simulink library "AEMS_Standard_Library"  (R2016b)
settings: Solver=ode45  StartTime=0.0  StopTime=10.0  RelTol=1e-3
undefined symbols (not defined in the file or in its folder): BkPY, carto, Cbx_extegr, Cbx_lpegrsys, Cbx_portegr, Cnx_bnk_nr_conf, Cnx_cyl_nr_conf, ConfigManagement, configuration_management, Cxx_dcm_io_tmr_end_xxxx, Cxx_dcm_rt_tmr_end, Cxx_DID_xxxx_IO_max, Cxx_DID_xxxx_IO_min, Cxx_egrhsofs, Cxx_vmaniegi, DEM_DEBOUNCE_FREEZE, DEM_DTR_CTL_INVISIBLE, DEM_DTR_CTL_NORMAL, Dem_DtrId2_XXX, Dem_DtrId3_XXX, Dem_DtrId4_XXX, Dem_DtrId5_XXX, Dem_DtrId6_XXX, Dem_DtrId7_XXX, Dem_DtrId8_XXX, Dem_DtrId9_XXX, Dem_DtrId_XXX, Dem_EnableConditionId2_XXX, Dem_EnableConditionId3_XXX, Dem_EnableConditionId4_XXX, Dem_EnableConditionId5_XXX, Dem_EnableConditionId6_XXX, Dem_EnableConditionId7_XXX, Dem_EnableConditionId8_XXX, Dem_EnableConditionId_XXX, Dem_EventId, Dem_EventId2_XXX, Dem_EventId3_XXX, Dem_EventId4_XXX, Dem_EventId5_XXX, Dem_EventId6_XXX, Dem_EventId7_XXX, Dem_EventId8_XXX, Dem_EventId9_XXX, Dem_EventId_Device_Faulttype, Dem_EventId_XXX, DEM_IUMPR_GENERAL_DENOMINATOR, DEM_OPCYC_IGNITION, Dem_RatioId2_XXX, Dem_RatioId3_XXX, Dem_RatioId4_XXX, Dem_RatioId5_XXX, Dem_RatioId6_XXX, Dem_RatioId7_XXX, Dem_RatioId8_XXX, Dem_RatioId_XXX, Dem_StorageConditionId2_XXX, Dem_StorageConditionId3_XXX, Dem_StorageConditionId4_XXX, Dem_StorageConditionId5_XXX ... (+65)
libraries: AEMS_Standard_Library x477, simulink x2
(part 32 of 39)

== system AEMS_Standard_Library/SUB/AEMS_DEM_SET_DTR_2DU/Dem_SetDTR_Call1 ==
  testresult1 : Inport  Interpolate=off
  lowerlimit1 : Inport  Port=2  Interpolate=off
  upperlimit1 : Inport  Port=3  Interpolate=off
  ctrl_flag1 : Inport  Port=4  Interpolate=off
  set_flag1 : EnablePort
      settings: AttributesFormatString=<states=%<StatesWhenEnabling>>
  AEMS_DEM_SETDTR1 : AEMS_Standard_Library/SUB/AEMS_DEM_SETDTR
      settings: AttributesFormatString=%<MaskType>
  Ctrlval_block1 : Constant  Value=DEM_DTR_CTL_NORMAL  OutDataTypeStr=uint8
  Ctrlval_block2 : Constant  Value=DEM_DTR_CTL_INVISIBLE  OutDataTypeStr=uint8
  DTRId_block1 : Constant  Value=Dem_DtrId_XXX  OutDataTypeStr=uint16
  Data Type Conversion : DataTypeConversion  OutDataTypeStr=int32  SaturateOnIntegerOverflow=on
  Data Type Conversion1 : DataTypeConversion  OutDataTypeStr=int32  SaturateOnIntegerOverflow=on
  Data Type Conversion2 : DataTypeConversion  OutDataTypeStr=int32  SaturateOnIntegerOverflow=on
  Limitter1 : Saturate  UpperLimit=1  LowerLimit=0
      settings: AttributesFormatString=<limits=%<UpperLimit>/%<LowerLimit>>
  Limitter2 : Saturate  UpperLimit=1  LowerLimit=0
      settings: AttributesFormatString=<limits=%<UpperLimit>/%<LowerLimit>>
  Limitter3 : Saturate  UpperLimit=1  LowerLimit=0
      settings: AttributesFormatString=<limits=%<UpperLimit>/%<LowerLimit>>
  Sum : Sum  OutDataTypeStr=Inherit: Inherit via back propagation  SaturateOnIntegerOverflow=on  InputSameDT=on
  Sum1 : Sum  OutDataTypeStr=Inherit: Inherit via back propagation  SaturateOnIntegerOverflow=on  InputSameDT=on
  Sum2 : Sum  OutDataTypeStr=Inherit: Inherit via back propagation  SaturateOnIntegerOverflow=on  InputSameDT=on
  Switch : Switch  Criteria=u2 ~= 0  ZeroCross=off  InputSameDT=on
      settings: AttributesFormatString=Criteria=%<Criteria>
  offset1 : Constant  Value=0  OutDataTypeStr=uint16
  offset2 : Constant  Value=0  OutDataTypeStr=uint16
  offset3 : Constant  Value=0  OutDataTypeStr=uint16
  wires:
  Switch/1 -> AEMS_DEM_SETDTR1/5  "ctrlval1"
  Ctrlval_block2/1 -> Switch/3
  ctrl_flag1/1 -> Switch/2
  Ctrlval_block1/1 -> Switch/1
  offset1/1 -> Sum/1
  Limitter1/1 -> Sum/2
  offset2/1 -> Sum1/1
  Limitter2/1 -> Sum1/2
  offset3/1 -> Sum2/1
  Limitter3/1 -> Sum2/2
  Sum/1 -> Data Type Conversion/1
  Sum1/1 -> Data Type Conversion1/1
  Sum2/1 -> Data Type Conversion2/1
  testresult1/1 -> Limitter1/1
  lowerlimit1/1 -> Limitter2/1
  upperlimit1/1 -> Limitter3/1
  Data Type Conversion/1 -> AEMS_DEM_SETDTR1/2  "result1"
  DTRId_block1/1 -> AEMS_DEM_SETDTR1/1  "dtrid1"
  Data Type Conversion1/1 -> AEMS_DEM_SETDTR1/3  "lowlimit1"
  Data Type Conversion2/1 -> AEMS_DEM_SETDTR1/4  "uplimit1"

== system AEMS_Standard_Library/SUB/AEMS_DEM_SET_DTR_2DU/Dem_SetDTR_Call2 ==
  testresult2 : Inport  Interpolate=off
  lowerlimit2 : Inport  Port=2  Interpolate=off
  upperlimit2 : Inport  Port=3  Interpolate=off
  ctrl_flag2 : Inport  Port=4  Interpolate=off
  set_flag2 : EnablePort
      settings: AttributesFormatString=<states=%<StatesWhenEnabling>>
  AEMS_DEM_SETDTR2 : AEMS_Standard_Library/SUB/AEMS_DEM_SETDTR
      settings: AttributesFormatString=%<MaskType>
  Ctrlval_block1 : Constant  Value=DEM_DTR_CTL_NORMAL  OutDataTypeStr=uint8
  Ctrlval_block2 : Constant  Value=DEM_DTR_CTL_INVISIBLE  OutDataTypeStr=uint8
  DTRId_block2 : Constant  Value=Dem_DtrId2_XXX  OutDataTypeStr=uint16
  Data Type Conversion3 : DataTypeConversion  OutDataTypeStr=int32  SaturateOnIntegerOverflow=on
  Data Type Conversion4 : DataTypeConversion  OutDataTypeStr=int32  SaturateOnIntegerOverflow=on
  Data Type Conversion5 : DataTypeConversion  OutDataTypeStr=int32  SaturateOnIntegerOverflow=on
  Limitter4 : Saturate  UpperLimit=1  LowerLimit=0
      settings: AttributesFormatString=<limits=%<UpperLimit>/%<LowerLimit>>
  Limitter5 : Saturate  UpperLimit=1  LowerLimit=0
      settings: AttributesFormatString=<limits=%<UpperLimit>/%<LowerLimit>>
  Limitter6 : Saturate  UpperLimit=1  LowerLimit=0
      settings: AttributesFormatString=<limits=%<UpperLimit>/%<LowerLimit>>
  Sum3 : Sum  OutDataTypeStr=Inherit: Inherit via back propagation  SaturateOnIntegerOverflow=on  InputSameDT=on
  Sum4 : Sum  OutDataTypeStr=Inherit: Inherit via back propagation  SaturateOnIntegerOverflow=on  InputSameDT=on
  Sum5 : Sum  OutDataTypeStr=Inherit: Inherit via back propagation  SaturateOnIntegerOverflow=on  InputSameDT=on
  Switch : Switch  Criteria=u2 ~= 0  ZeroCross=off  InputSameDT=on
      settings: AttributesFormatString=Criteria=%<Criteria>
  offset4 : Constant  Value=0  OutDataTypeStr=uint16
  offset5 : Constant  Value=0  OutDataTypeStr=uint16
  offset6 : Constant  Value=0  OutDataTypeStr=uint16
  wires:
  Ctrlval_block1/1 -> Switch/1
  Switch/1 -> AEMS_DEM_SETDTR2/5  "ctrlval2"
  Ctrlval_block2/1 -> Switch/3
  ctrl_flag2/1 -> Switch/2
  offset4/1 -> Sum3/1
  Limitter4/1 -> Sum3/2
  offset5/1 -> Sum4/1
  Limitter5/1 -> Sum4/2
  offset6/1 -> Sum5/1
  Limitter6/1 -> Sum5/2
  Sum3/1 -> Data Type Conversion3/1
  Sum4/1 -> Data Type Conversion4/1
  Sum5/1 -> Data Type Conversion5/1
  testresult2/1 -> Limitter4/1
  lowerlimit2/1 -> Limitter5/1
  upperlimit2/1 -> Limitter6/1
  DTRId_block2/1 -> AEMS_DEM_SETDTR2/1  "dtrid2"
  Data Type Conversion3/1 -> AEMS_DEM_SETDTR2/2  "result2"
  Data Type Conversion4/1 -> AEMS_DEM_SETDTR2/3  "lowlimit2"
  Data Type Conversion5/1 -> AEMS_DEM_SETDTR2/4  "uplimit2"

== system AEMS_Standard_Library/SUB/AEMS_DEM_SET_DTR_8DS/Deadzone ==
  testresult : Inport  Interpolate=off
  lowerlimit : Inport  Port=2  Interpolate=off
  upperlimit : Inport  Port=3  Interpolate=off
  Sum1 : Sum  Inputs=-+  OutDataTypeStr=Inherit: Inherit via back propagation  InputSameDT=on
  Sum3 : Sum  OutDataTypeStr=Inherit: Inherit via back propagation  SaturateOnIntegerOverflow=on  InputSameDT=on
  Switch{,1,3..4} (4 alike) : Switch  Criteria=u2 ~= 0  ZeroCross=off  InputSameDT=on
      settings: AttributesFormatString=Criteria=%<Criteria>
  relational2 : RelationalOperator  DisableCoverage=on  OutDataTypeStr=boolean  ZeroCross=off  RndMeth=Nearest  InputSameDT=on
  relational3 : RelationalOperator  DisableCoverage=on  Operator=<  OutDataTypeStr=boolean  ZeroCross=off  RndMeth=Nearest  InputSameDT=on
  relational4 : RelationalOperator  DisableCoverage=on  OutDataTypeStr=boolean  ZeroCross=off  RndMeth=Nearest  InputSameDT=on
  relational5 : RelationalOperator  DisableCoverage=on  Operator=<=  OutDataTypeStr=boolean  ZeroCross=off  RndMeth=Nearest  InputSameDT=on
  resolution_block1 : Constant  OutDataTypeStr=single
  resolution_block2 : Constant  OutDataTypeStr=single
  customresult : Outport
  wires:
  Switch/1 -> customresult/1  "customresult"
  Sum3/1 -> Switch1/1, relational2/2
  Switch4/1 -> Switch3/3
  Switch1/1 -> Switch/3
  lowerlimit/1 -> relational4/2, Sum1/2
  relational5/1 -> Switch4/2
  relational4/1 -> Switch3/2
  relational3/1 -> Switch1/2
  resolution_block1/1 -> Sum3/2
  upperlimit/1 -> Sum3/1, relational3/1
  relational2/1 -> Switch/2
  testresult/1 -> Switch/1, relational2/1, relational4/1, Switch3/1, Switch4/3, relational5/2, relational3/2
  Switch3/1 -> Switch1/3
  Sum1/1 -> relational5/1, Switch4/1
  resolution_block2/1 -> Sum1/1

== system AEMS_Standard_Library/SUB/AEMS_DEM_SET_DTR_8DS/Dem_SetDTR_Call1 ==
  customresult1 : Inport  Interpolate=off
  lowerlimit1 : Inport  Port=2  Interpolate=off
  upperlimit1 : Inport  Port=3  Interpolate=off
  ctrl_flag1 : Inport  Port=4  Interpolate=off
  set_flag1 : EnablePort
      settings: AttributesFormatString=<states=%<StatesWhenEnabling>>
  AEMS_DEM_SETDTR1 : AEMS_Standard_Library/SUB/AEMS_DEM_SETDTR  Tag=[LIB]
      settings: AttributesFormatString=%<MaskType>
  Ctrlval_block1 : Constant  Value=DEM_DTR_CTL_NORMAL  OutDataTypeStr=uint8
  Ctrlval_block2 : Constant  Value=DEM_DTR_CTL_INVISIBLE  OutDataTypeStr=uint8
  DTRId_block1 : Constant  Value=Dem_DtrId_XXX  OutDataTypeStr=uint16
  Data Type Conversion : DataTypeConversion  OutDataTypeStr=int32  SaturateOnIntegerOverflow=on
  Data Type Conversion1 : DataTypeConversion  OutDataTypeStr=int32  SaturateOnIntegerOverflow=on
  Data Type Conversion2 : DataTypeConversion  OutDataTypeStr=int32  SaturateOnIntegerOverflow=on
  Divide1 : Product  Inputs=*/  OutDataTypeStr=Inherit: Inherit via back propagation  SaturateOnIntegerOverflow=on
  Divide2 : Product  Inputs=*/  OutDataTypeStr=Inherit: Inherit via back propagation  SaturateOnIntegerOverflow=on
  Divide3 : Product  Inputs=*/  OutDataTypeStr=Inherit: Inherit via back propagation  SaturateOnIntegerOverflow=on
  Limitter1 : Saturate  UpperLimit=1  LowerLimit=0
      settings: AttributesFormatString=<limits=%<UpperLimit>/%<LowerLimit>>
  Limitter2 : Saturate  UpperLimit=1  LowerLimit=0
      settings: AttributesFormatString=<limits=%<UpperLimit>/%<LowerLimit>>
  Limitter3 : Saturate  UpperLimit=1  LowerLimit=0
      settings: AttributesFormatString=<limits=%<UpperLimit>/%<LowerLimit>>
  Resolution_block1 : Constant  OutDataTypeStr=single
  Resolution_block2 : Constant  OutDataTypeStr=single
  Resolution_block3 : Constant  OutDataTypeStr=single
  Switch : Switch  Criteria=u2 ~= 0  ZeroCross=off  InputSameDT=on
      settings: AttributesFormatString=Criteria=%<Criteria>
  wires:
  DTRId_block1/1 -> AEMS_DEM_SETDTR1/1  "dtrid1"
  Resolution_block1/1 -> Divide1/2
  Limitter1/1 -> Divide1/1
  Limitter3/1 -> Divide3/1
  customresult1/1 -> Limitter1/1
  lowerlimit1/1 -> Limitter2/1
  upperlimit1/1 -> Limitter3/1
  Data Type Conversion1/1 -> AEMS_DEM_SETDTR1/3  "lowlimit1"
  Data Type Conversion2/1 -> AEMS_DEM_SETDTR1/4  "uplimit1"
  Data Type Conversion/1 -> AEMS_DEM_SETDTR1/2  "result1"
  Limitter2/1 -> Divide2/1
  Resolution_block2/1 -> Divide2/2
  Resolution_block3/1 -> Divide3/2
  Switch/1 -> AEMS_DEM_SETDTR1/5  "ctrlval1"
  Ctrlval_block1/1 -> Switch/1
  ctrl_flag1/1 -> Switch/2
  Ctrlval_block2/1 -> Switch/3
  Divide1/1 -> Data Type Conversion/1
  Divide2/1 -> Data Type Conversion1/1
  Divide3/1 -> Data Type Conversion2/1

== system AEMS_Standard_Library/SUB/AEMS_DEM_SET_DTR_8DS/Dem_SetDTR_Call2 ==
  customresult2 : Inport  Interpolate=off
  lowerlimit2 : Inport  Port=2  Interpolate=off
  upperlimit2 : Inport  Port=3  Interpolate=off
  ctrl_flag2 : Inport  Port=4  Interpolate=off
  set_flag2 : EnablePort
      settings: AttributesFormatString=<states=%<StatesWhenEnabling>>
  AEMS_DEM_SETDTR2 : AEMS_Standard_Library/SUB/AEMS_DEM_SETDTR  Tag=[LIB]
      settings: AttributesFormatString=%<MaskType>
  Ctrlval_block1 : Constant  Value=DEM_DTR_CTL_NORMAL  OutDataTypeStr=uint8
  Ctrlval_block2 : Constant  Value=DEM_DTR_CTL_INVISIBLE  OutDataTypeStr=uint8
  DTRId_block2 : Constant  Value=Dem_DtrId2_XXX  OutDataTypeStr=uint16
  Data Type Conversion : DataTypeConversion  OutDataTypeStr=int32  SaturateOnIntegerOverflow=on
  Data Type Conversion1 : DataTypeConversion  OutDataTypeStr=int32  SaturateOnIntegerOverflow=on
  Data Type Conversion2 : DataTypeConversion  OutDataTypeStr=int32  SaturateOnIntegerOverflow=on
  Divide1 : Product  Inputs=*/  OutDataTypeStr=Inherit: Inherit via back propagation  SaturateOnIntegerOverflow=on
  Divide2 : Product  Inputs=*/  OutDataTypeStr=Inherit: Inherit via back propagation  SaturateOnIntegerOverflow=on
  Divide3 : Product  Inputs=*/  OutDataTypeStr=Inherit: Inherit via back propagation  SaturateOnIntegerOverflow=on
  Limitter4 : Saturate  UpperLimit=1  LowerLimit=0
      settings: AttributesFormatString=<limits=%<UpperLimit>/%<LowerLimit>>
  Limitter5 : Saturate  UpperLimit=1  LowerLimit=0
      settings: AttributesFormatString=<limits=%<UpperLimit>/%<LowerLimit>>
  Limitter6 : Saturate  UpperLimit=1  LowerLimit=0
      settings: AttributesFormatString=<limits=%<UpperLimit>/%<LowerLimit>>
  Resolution_block4 : Constant  OutDataTypeStr=single
  Resolution_block5 : Constant  OutDataTypeStr=single
  Resolution_block6 : Constant  OutDataTypeStr=single
  Switch : Switch  Criteria=u2 ~= 0  ZeroCross=off  InputSameDT=on
      settings: AttributesFormatString=Criteria=%<Criteria>
  wires:
  DTRId_block2/1 -> AEMS_DEM_SETDTR2/1  "dtrid2"
  Resolution_block4/1 -> Divide1/2
  Limitter4/1 -> Divide1/1
  Limitter6/1 -> Divide3/1
  customresult2/1 -> Limitter4/1
  lowerlimit2/1 -> Limitter5/1
  upperlimit2/1 -> Limitter6/1
  Data Type Conversion1/1 -> AEMS_DEM_SETDTR2/3  "lowlimit2"
  Data Type Conversion2/1 -> AEMS_DEM_SETDTR2/4  "uplimit2"
  Data Type Conversion/1 -> AEMS_DEM_SETDTR2/2  "result2"
  Limitter5/1 -> Divide2/1
  Resolution_block5/1 -> Divide2/2
  Resolution_block6/1 -> Divide3/2
  Divide1/1 -> Data Type Conversion/1
  Divide2/1 -> Data Type Conversion1/1
  Divide3/1 -> Data Type Conversion2/1
  Switch/1 -> AEMS_DEM_SETDTR2/5  "ctrlval2"
  Ctrlval_block1/1 -> Switch/1
  ctrl_flag2/1 -> Switch/2
  Ctrlval_block2/1 -> Switch/3

== system AEMS_Standard_Library/SUB/AEMS_DEM_SET_DTR_8DS/Dem_SetDTR_Call3 ==
  customresult3 : Inport  Interpolate=off
  lowerlimit3 : Inport  Port=2  Interpolate=off
  upperlimit3 : Inport  Port=3  Interpolate=off
  ctrl_flag3 : Inport  Port=4  Interpolate=off
  set_flag3 : EnablePort
      settings: AttributesFormatString=<states=%<StatesWhenEnabling>>
  AEMS_DEM_SETDTR3 : AEMS_Standard_Library/SUB/AEMS_DEM_SETDTR  Tag=[LIB]
      settings: AttributesFormatString=%<MaskType>
  Ctrlval_block1 : Constant  Value=DEM_DTR_CTL_NORMAL  OutDataTypeStr=uint8
  Ctrlval_block2 : Constant  Value=DEM_DTR_CTL_INVISIBLE  OutDataTypeStr=uint8
  DTRId_block3 : Constant  Value=Dem_DtrId3_XXX  OutDataTypeStr=uint16
  Data Type Conversion : DataTypeConversion  OutDataTypeStr=int32  SaturateOnIntegerOverflow=on
  Data Type Conversion1 : DataTypeConversion  OutDataTypeStr=int32  SaturateOnIntegerOverflow=on
  Data Type Conversion2 : DataTypeConversion  OutDataTypeStr=int32  SaturateOnIntegerOverflow=on
  Divide1 : Product  Inputs=*/  OutDataTypeStr=Inherit: Inherit via back propagation  SaturateOnIntegerOverflow=on
  Divide2 : Product  Inputs=*/  OutDataTypeStr=Inherit: Inherit via back propagation  SaturateOnIntegerOverflow=on
  Divide3 : Product  Inputs=*/  OutDataTypeStr=Inherit: Inherit via back propagation  SaturateOnIntegerOverflow=on
  Limitter7 : Saturate  UpperLimit=1  LowerLimit=0
      settings: AttributesFormatString=<limits=%<UpperLimit>/%<LowerLimit>>
  Limitter8 : Saturate  UpperLimit=1  LowerLimit=0
      settings: AttributesFormatString=<limits=%<UpperLimit>/%<LowerLimit>>
  Limitter9 : Saturate  UpperLimit=1  LowerLimit=0
      settings: AttributesFormatString=<limits=%<UpperLimit>/%<LowerLimit>>
  Resolution_block7 : Constant  OutDataTypeStr=single
  Resolution_block8 : Constant  OutDataTypeStr=single
  Resolution_block9 : Constant  OutDataTypeStr=single
  Switch : Switch  Criteria=u2 ~= 0  ZeroCross=off  InputSameDT=on
      settings: AttributesFormatString=Criteria=%<Criteria>
  wires:
  DTRId_block3/1 -> AEMS_DEM_SETDTR3/1  "dtrid3"
  Resolution_block7/1 -> Divide1/2
  Limitter7/1 -> Divide1/1
  Limitter9/1 -> Divide3/1
  customresult3/1 -> Limitter7/1
  lowerlimit3/1 -> Limitter8/1
  upperlimit3/1 -> Limitter9/1
  Data Type Conversion1/1 -> AEMS_DEM_SETDTR3/3  "lowlimit3"
  Data Type Conversion2/1 -> AEMS_DEM_SETDTR3/4  "uplimit3"
  Data Type Conversion/1 -> AEMS_DEM_SETDTR3/2  "result3"
  Limitter8/1 -> Divide2/1
  Resolution_block8/1 -> Divide2/2
  Resolution_block9/1 -> Divide3/2
  Divide1/1 -> Data Type Conversion/1
  Divide2/1 -> Data Type Conversion1/1
  Divide3/1 -> Data Type Conversion2/1
  Switch/1 -> AEMS_DEM_SETDTR3/5  "ctrlval3"
  Ctrlval_block1/1 -> Switch/1
  ctrl_flag3/1 -> Switch/2
  Ctrlval_block2/1 -> Switch/3

== system AEMS_Standard_Library/SUB/AEMS_DEM_SET_DTR_8DS/Dem_SetDTR_Call4 ==
  customresult4 : Inport  Interpolate=off
  lowerlimit4 : Inport  Port=2  Interpolate=off
  upperlimit4 : Inport  Port=3  Interpolate=off
  ctrl_flag4 : Inport  Port=4  Interpolate=off
  set_flag4 : EnablePort
      settings: AttributesFormatString=<states=%<StatesWhenEnabling>>
  AEMS_DEM_SETDTR4 : AEMS_Standard_Library/SUB/AEMS_DEM_SETDTR  Tag=[LIB]
      settings: AttributesFormatString=%<MaskType>
  Ctrlval_block1 : Constant  Value=DEM_DTR_CTL_NORMAL  OutDataTypeStr=uint8
  Ctrlval_block2 : Constant  Value=DEM_DTR_CTL_INVISIBLE  OutDataTypeStr=uint8
  DTRId_block4 : Constant  Value=Dem_DtrId4_XXX  OutDataTypeStr=uint16
  Data Type Conversion : DataTypeConversion  OutDataTypeStr=int32  SaturateOnIntegerOverflow=on
  Data Type Conversion1 : DataTypeConversion  OutDataTypeStr=int32  SaturateOnIntegerOverflow=on
  Data Type Conversion2 : DataTypeConversion  OutDataTypeStr=int32  SaturateOnIntegerOverflow=on
  Divide1 : Product  Inputs=*/  OutDataTypeStr=Inherit: Inherit via back propagation  SaturateOnIntegerOverflow=on
  Divide2 : Product  Inputs=*/  OutDataTypeStr=Inherit: Inherit via back propagation  SaturateOnIntegerOverflow=on
  Divide3 : Product  Inputs=*/  OutDataTypeStr=Inherit: Inherit via back propagation  SaturateOnIntegerOverflow=on
  Limitter10 : Saturate  UpperLimit=1  LowerLimit=0
      settings: AttributesFormatString=<limits=%<UpperLimit>/%<LowerLimit>>
  Limitter11 : Saturate  UpperLimit=1  LowerLimit=0
      settings: AttributesFormatString=<limits=%<UpperLimit>/%<LowerLimit>>
  Limitter12 : Saturate  UpperLimit=1  LowerLimit=0
      settings: AttributesFormatString=<limits=%<UpperLimit>/%<LowerLimit>>
  Resolution_block10 : Constant  OutDataTypeStr=single
  Resolution_block11 : Constant  OutDataTypeStr=single
  Resolution_block12 : Constant  OutDataTypeStr=single
  Switch : Switch  Criteria=u2 ~= 0  ZeroCross=off  InputSameDT=on
      settings: AttributesFormatString=Criteria=%<Criteria>
  wires:
  DTRId_block4/1 -> AEMS_DEM_SETDTR4/1  "dtrid4"
  Resolution_block10/1 -> Divide1/2
  Limitter10/1 -> Divide1/1
  Limitter12/1 -> Divide3/1
  customresult4/1 -> Limitter10/1
  lowerlimit4/1 -> Limitter11/1
  upperlimit4/1 -> Limitter12/1
  Data Type Conversion1/1 -> AEMS_DEM_SETDTR4/3  "lowlimit4"
  Data Type Conversion2/1 -> AEMS_DEM_SETDTR4/4  "uplimit4"
  Data Type Conversion/1 -> AEMS_DEM_SETDTR4/2  "result4"
  Limitter11/1 -> Divide2/1
  Resolution_block11/1 -> Divide2/2
  Resolution_block12/1 -> Divide3/2
  Ctrlval_block1/1 -> Switch/1
  ctrl_flag4/1 -> Switch/2
  Ctrlval_block2/1 -> Switch/3
  Switch/1 -> AEMS_DEM_SETDTR4/5  "ctrlval4"
  Divide3/1 -> Data Type Conversion2/1
  Divide2/1 -> Data Type Conversion1/1
  Divide1/1 -> Data Type Conversion/1

== system AEMS_Standard_Library/SUB/AEMS_DEM_SET_DTR_8DS/Dem_SetDTR_Call5 ==
  customresult5 : Inport  Interpolate=off
  lowerlimit5 : Inport  Port=2  Interpolate=off
  upperlimit5 : Inport  Port=3  Interpolate=off
  ctrl_flag5 : Inport  Port=4  Interpolate=off
  set_flag5 : EnablePort
      settings: AttributesFormatString=<states=%<StatesWhenEnabling>>
  AEMS_DEM_SETDTR5 : AEMS_Standard_Library/SUB/AEMS_DEM_SETDTR  Tag=[LIB]
      settings: AttributesFormatString=%<MaskType>
  Ctrlval_block1 : Constant  Value=DEM_DTR_CTL_NORMAL  OutDataTypeStr=uint8
  Ctrlval_block2 : Constant  Value=DEM_DTR_CTL_INVISIBLE  OutDataTypeStr=uint8
  DTRId_block5 : Constant  Value=Dem_DtrId5_XXX  OutDataTypeStr=uint16
  Data Type Conversion : DataTypeConversion  OutDataTypeStr=int32  SaturateOnIntegerOverflow=on
  Data Type Conversion1 : DataTypeConversion  OutDataTypeStr=int32  SaturateOnIntegerOverflow=on
  Data Type Conversion2 : DataTypeConversion  OutDataTypeStr=int32  SaturateOnIntegerOverflow=on
  Divide1 : Product  Inputs=*/  OutDataTypeStr=Inherit: Inherit via back propagation  SaturateOnIntegerOverflow=on
  Divide2 : Product  Inputs=*/  OutDataTypeStr=Inherit: Inherit via back propagation  SaturateOnIntegerOverflow=on
  Divide3 : Product  Inputs=*/  OutDataTypeStr=Inherit: Inherit via back propagation  SaturateOnIntegerOverflow=on
  Limitter13 : Saturate  UpperLimit=1  LowerLimit=0
      settings: AttributesFormatString=<limits=%<UpperLimit>/%<LowerLimit>>
  Limitter14 : Saturate  UpperLimit=1  LowerLimit=0
      settings: AttributesFormatString=<limits=%<UpperLimit>/%<LowerLimit>>
  Limitter15 : Saturate  UpperLimit=1  LowerLimit=0
      settings: AttributesFormatString=<limits=%<UpperLimit>/%<LowerLimit>>
  Resolution_block13 : Constant  OutDataTypeStr=single
  Resolution_block14 : Constant  OutDataTypeStr=single
  Resolution_block15 : Constant  OutDataTypeStr=single
  Switch : Switch  Criteria=u2 ~= 0  ZeroCross=off  InputSameDT=on
      settings: AttributesFormatString=Criteria=%<Criteria>
  wires:
  DTRId_block5/1 -> AEMS_DEM_SETDTR5/1  "dtrid5"
  Resolution_block13/1 -> Divide1/2
  Limitter13/1 -> Divide1/1
  Limitter15/1 -> Divide3/1
  customresult5/1 -> Limitter13/1
  lowerlimit5/1 -> Limitter14/1
  upperlimit5/1 -> Limitter15/1
  Data Type Conversion1/1 -> AEMS_DEM_SETDTR5/3  "lowlimit5"
  Switch/1 -> AEMS_DEM_SETDTR5/5  "ctrlval5"
  Data Type Conversion2/1 -> AEMS_DEM_SETDTR5/4  "uplimit5"
  Data Type Conversion/1 -> AEMS_DEM_SETDTR5/2  "result5"
  Limitter14/1 -> Divide2/1
  Resolution_block14/1 -> Divide2/2
  Resolution_block15/1 -> Divide3/2
  Divide1/1 -> Data Type Conversion/1
  Divide2/1 -> Data Type Conversion1/1
  Divide3/1 -> Data Type Conversion2/1
  Ctrlval_block1/1 -> Switch/1
  ctrl_flag5/1 -> Switch/2
  Ctrlval_block2/1 -> Switch/3

== system AEMS_Standard_Library/SUB/AEMS_DEM_SET_DTR_8DS/Dem_SetDTR_Call6 ==
  customresult6 : Inport  Interpolate=off
  lowerlimit6 : Inport  Port=2  Interpolate=off
  upperlimit6 : Inport  Port=3  Interpolate=off
  ctrl_flag6 : Inport  Port=4  Interpolate=off
  set_flag6 : EnablePort
      settings: AttributesFormatString=<states=%<StatesWhenEnabling>>
  AEMS_DEM_SETDTR6 : AEMS_Standard_Library/SUB/AEMS_DEM_SETDTR  Tag=[LIB]
      settings: AttributesFormatString=%<MaskType>
  Ctrlval_block1 : Constant  Value=DEM_DTR_CTL_NORMAL  OutDataTypeStr=uint8
  Ctrlval_block2 : Constant  Value=DEM_DTR_CTL_INVISIBLE  OutDataTypeStr=uint8
  DTRId_block6 : Constant  Value=Dem_DtrId6_XXX  OutDataTypeStr=uint16
  Data Type Conversion : DataTypeConversion  OutDataTypeStr=int32  SaturateOnIntegerOverflow=on
  Data Type Conversion1 : DataTypeConversion  OutDataTypeStr=int32  SaturateOnIntegerOverflow=on
  Data Type Conversion2 : DataTypeConversion  OutDataTypeStr=int32  SaturateOnIntegerOverflow=on
  Divide1 : Product  Inputs=*/  OutDataTypeStr=Inherit: Inherit via back propagation  SaturateOnIntegerOverflow=on
  Divide2 : Product  Inputs=*/  OutDataTypeStr=Inherit: Inherit via back propagation  SaturateOnIntegerOverflow=on
  Divide3 : Product  Inputs=*/  OutDataTypeStr=Inherit: Inherit via back propagation  SaturateOnIntegerOverflow=on
  Limitter16 : Saturate  UpperLimit=1  LowerLimit=0
      settings: AttributesFormatString=<limits=%<UpperLimit>/%<LowerLimit>>
  Limitter17 : Saturate  UpperLimit=1  LowerLimit=0
      settings: AttributesFormatString=<limits=%<UpperLimit>/%<LowerLimit>>
  Limitter18 : Saturate  UpperLimit=1  LowerLimit=0
      settings: AttributesFormatString=<limits=%<UpperLimit>/%<LowerLimit>>
  Resolution_block16 : Constant  OutDataTypeStr=single
  Resolution_block17 : Constant  OutDataTypeStr=single
  Resolution_block18 : Constant  OutDataTypeStr=single
  Switch : Switch  Criteria=u2 ~= 0  ZeroCross=off  InputSameDT=on
      settings: AttributesFormatString=Criteria=%<Criteria>
  wires:
  DTRId_block6/1 -> AEMS_DEM_SETDTR6/1  "dtrid6"
  Resolution_block16/1 -> Divide1/2
  Limitter16/1 -> Divide1/1
  Limitter18/1 -> Divide3/1
  customresult6/1 -> Limitter16/1
  lowerlimit6/1 -> Limitter17/1
  upperlimit6/1 -> Limitter18/1
  Data Type Conversion1/1 -> AEMS_DEM_SETDTR6/3  "lowlimit6"
  Switch/1 -> AEMS_DEM_SETDTR6/5  "ctrlval6"
  Data Type Conversion2/1 -> AEMS_DEM_SETDTR6/4  "uplimit6"
  Data Type Conversion/1 -> AEMS_DEM_SETDTR6/2  "result6"
  Limitter17/1 -> Divide2/1
  Resolution_block17/1 -> Divide2/2
  Resolution_block18/1 -> Divide3/2
  Ctrlval_block1/1 -> Switch/1
  ctrl_flag6/1 -> Switch/2
  Ctrlval_block2/1 -> Switch/3
  Divide3/1 -> Data Type Conversion2/1
  Divide2/1 -> Data Type Conversion1/1
  Divide1/1 -> Data Type Conversion/1

== system AEMS_Standard_Library/SUB/AEMS_DEM_SET_DTR_8DS/Dem_SetDTR_Call7 ==
  customresult7 : Inport  Interpolate=off
  lowerlimit7 : Inport  Port=2  Interpolate=off
  upperlimit7 : Inport  Port=3  Interpolate=off
  ctrl_flag7 : Inport  Port=4  Interpolate=off
  set_flag7 : EnablePort
      settings: AttributesFormatString=<states=%<StatesWhenEnabling>>
  AEMS_DEM_SETDTR7 : AEMS_Standard_Library/SUB/AEMS_DEM_SETDTR  Tag=[LIB]
      settings: AttributesFormatString=%<MaskType>
  Ctrlval_block1 : Constant  Value=DEM_DTR_CTL_NORMAL  OutDataTypeStr=uint8
  Ctrlval_block2 : Constant  Value=DEM_DTR_CTL_INVISIBLE  OutDataTypeStr=uint8
  DTRId_block7 : Constant  Value=Dem_DtrId7_XXX  OutDataTypeStr=uint16
  Data Type Conversion : DataTypeConversion  OutDataTypeStr=int32  SaturateOnIntegerOverflow=on
  Data Type Conversion1 : DataTypeConversion  OutDataTypeStr=int32  SaturateOnIntegerOverflow=on
  Data Type Conversion2 : DataTypeConversion  OutDataTypeStr=int32  SaturateOnIntegerOverflow=on
  Divide1 : Product  Inputs=*/  OutDataTypeStr=Inherit: Inherit via back propagation  SaturateOnIntegerOverflow=on
  Divide2 : Product  Inputs=*/  OutDataTypeStr=Inherit: Inherit via back propagation  SaturateOnIntegerOverflow=on
  Divide3 : Product  Inputs=*/  OutDataTypeStr=Inherit: Inherit via back propagation  SaturateOnIntegerOverflow=on
  Limitter19 : Saturate  UpperLimit=1  LowerLimit=0
      settings: AttributesFormatString=<limits=%<UpperLimit>/%<LowerLimit>>
  Limitter20 : Saturate  UpperLimit=1  LowerLimit=0
      settings: AttributesFormatString=<limits=%<UpperLimit>/%<LowerLimit>>
  Limitter21 : Saturate  UpperLimit=1  LowerLimit=0
      settings: AttributesFormatString=<limits=%<UpperLimit>/%<LowerLimit>>
  Resolution_block19 : Constant  OutDataTypeStr=single
  Resolution_block20 : Constant  OutDataTypeStr=single
  Resolution_block21 : Constant  OutDataTypeStr=single
  Switch : Switch  Criteria=u2 ~= 0  ZeroCross=off  InputSameDT=on
      settings: AttributesFormatString=Criteria=%<Criteria>
  wires:
  DTRId_block7/1 -> AEMS_DEM_SETDTR7/1  "dtrid7"
  Resolution_block19/1 -> Divide1/2
  Limitter19/1 -> Divide1/1
  Limitter21/1 -> Divide3/1
  customresult7/1 -> Limitter19/1
  lowerlimit7/1 -> Limitter20/1
  upperlimit7/1 -> Limitter21/1
  Data Type Conversion1/1 -> AEMS_DEM_SETDTR7/3  "lowlimit7"
  Data Type Conversion2/1 -> AEMS_DEM_SETDTR7/4  "uplimit7"
  Data Type Conversion/1 -> AEMS_DEM_SETDTR7/2  "result7"
  Limitter20/1 -> Divide2/1
  Resolution_block20/1 -> Divide2/2
  Resolution_block21/1 -> Divide3/2
  Divide1/1 -> Data Type Conversion/1
  Divide2/1 -> Data Type Conversion1/1
  Divide3/1 -> Data Type Conversion2/1
  Switch/1 -> AEMS_DEM_SETDTR7/5  "ctrlval7"
  Ctrlval_block1/1 -> Switch/1
  ctrl_flag7/1 -> Switch/2
  Ctrlval_block2/1 -> Switch/3

== system AEMS_Standard_Library/SUB/AEMS_DEM_SET_DTR_8DS/Dem_SetDTR_Call8 ==
  customresult8 : Inport  Interpolate=off
  lowerlimit8 : Inport  Port=2  Interpolate=off
  upperlimit8 : Inport  Port=3  Interpolate=off
  ctrl_flag8 : Inport  Port=4  Interpolate=off
  set_flag8 : EnablePort
      settings: AttributesFormatString=<states=%<StatesWhenEnabling>>
  AEMS_DEM_SETDTR8 : AEMS_Standard_Library/SUB/AEMS_DEM_SETDTR  Tag=[LIB]
      settings: AttributesFormatString=%<MaskType>
  Ctrlval_block1 : Constant  Value=DEM_DTR_CTL_NORMAL  OutDataTypeStr=uint8
  Ctrlval_block2 : Constant  Value=DEM_DTR_CTL_INVISIBLE  OutDataTypeStr=uint8
  DTRId_block8 : Constant  Value=Dem_DtrId8_XXX  OutDataTypeStr=uint16
  Data Type Conversion : DataTypeConversion  OutDataTypeStr=int32  SaturateOnIntegerOverflow=on
  Data Type Conversion1 : DataTypeConversion  OutDataTypeStr=int32  SaturateOnIntegerOverflow=on
  Data Type Conversion2 : DataTypeConversion  OutDataTypeStr=int32  SaturateOnIntegerOverflow=on
  Divide1 : Product  Inputs=*/  OutDataTypeStr=Inherit: Inherit via back propagation  SaturateOnIntegerOverflow=on
  Divide2 : Product  Inputs=*/  OutDataTypeStr=Inherit: Inherit via back propagation  SaturateOnIntegerOverflow=on
  Divide3 : Product  Inputs=*/  OutDataTypeStr=Inherit: Inherit via back propagation  SaturateOnIntegerOverflow=on
  Limitter22 : Saturate  UpperLimit=1  LowerLimit=0
      settings: AttributesFormatString=<limits=%<UpperLimit>/%<LowerLimit>>
  Limitter23 : Saturate  UpperLimit=1  LowerLimit=0
      settings: AttributesFormatString=<limits=%<UpperLimit>/%<LowerLimit>>
  Limitter24 : Saturate  UpperLimit=1  LowerLimit=0
      settings: AttributesFormatString=<limits=%<UpperLimit>/%<LowerLimit>>
  Resolution_block22 : Constant  OutDataTypeStr=single
  Resolution_block23 : Constant  OutDataTypeStr=single
  Resolution_block24 : Constant  OutDataTypeStr=single
  Switch : Switch  Criteria=u2 ~= 0  ZeroCross=off  InputSameDT=on
      settings: AttributesFormatString=Criteria=%<Criteria>
  wires:
  DTRId_block8/1 -> AEMS_DEM_SETDTR8/1  "dtrid8"
  Resolution_block22/1 -> Divide1/2
  Limitter22/1 -> Divide1/1
  Limitter24/1 -> Divide3/1
  customresult8/1 -> Limitter22/1
  lowerlimit8/1 -> Limitter23/1
  upperlimit8/1 -> Limitter24/1
  Data Type Conversion1/1 -> AEMS_DEM_SETDTR8/3  "lowlimit8"
  Data Type Conversion2/1 -> AEMS_DEM_SETDTR8/4  "uplimit8"
  Data Type Conversion/1 -> AEMS_DEM_SETDTR8/2  "result8"
  Limitter23/1 -> Divide2/1
  Resolution_block23/1 -> Divide2/2
  Resolution_block24/1 -> Divide3/2
  Divide1/1 -> Data Type Conversion/1
  Divide2/1 -> Data Type Conversion1/1
  Divide3/1 -> Data Type Conversion2/1
  Switch/1 -> AEMS_DEM_SETDTR8/5  "ctrlval8"
  Ctrlval_block1/1 -> Switch/1
  ctrl_flag8/1 -> Switch/2
  Ctrlval_block2/1 -> Switch/3

== system AEMS_Standard_Library/SUB/AEMS_DEM_SET_DTR_8DU/Dem_SetDTR_Call1 ==
  testresult1 : Inport  Interpolate=off
  lowerlimit1 : Inport  Port=2  Interpolate=off
  upperlimit1 : Inport  Port=3  Interpolate=off
  ctrl_flag1 : Inport  Port=4  Interpolate=off
  set_flag1 : EnablePort
      settings: AttributesFormatString=<states=%<StatesWhenEnabling>>
  AEMS_DEM_SETDTR1 : AEMS_Standard_Library/SUB/AEMS_DEM_SETDTR  Tag=[LIB]
      settings: AttributesFormatString=%<MaskType>
  Ctrlval_block1 : Constant  Value=DEM_DTR_CTL_NORMAL  OutDataTypeStr=uint8
  Ctrlval_block2 : Constant  Value=DEM_DTR_CTL_INVISIBLE  OutDataTypeStr=uint8
  DTRId_block1 : Constant  Value=Dem_DtrId_XXX  OutDataTypeStr=uint16
  Data Type Conversion : DataTypeConversion  OutDataTypeStr=int32  SaturateOnIntegerOverflow=on
  Data Type Conversion1 : DataTypeConversion  OutDataTypeStr=int32  SaturateOnIntegerOverflow=on
  Data Type Conversion2 : DataTypeConversion  OutDataTypeStr=int32  SaturateOnIntegerOverflow=on
  Limitter1 : Saturate  UpperLimit=1  LowerLimit=0
      settings: AttributesFormatString=<limits=%<UpperLimit>/%<LowerLimit>>
  Limitter2 : Saturate  UpperLimit=1  LowerLimit=0
      settings: AttributesFormatString=<limits=%<UpperLimit>/%<LowerLimit>>
  Limitter3 : Saturate  UpperLimit=1  LowerLimit=0
      settings: AttributesFormatString=<limits=%<UpperLimit>/%<LowerLimit>>
  Sum : Sum  OutDataTypeStr=Inherit: Inherit via back propagation  SaturateOnIntegerOverflow=on  InputSameDT=on
  Sum1 : Sum  OutDataTypeStr=Inherit: Inherit via back propagation  SaturateOnIntegerOverflow=on  InputSameDT=on
  Sum2 : Sum  OutDataTypeStr=Inherit: Inherit via back propagation  SaturateOnIntegerOverflow=on  InputSameDT=on
  Switch : Switch  Criteria=u2 ~= 0  ZeroCross=off  InputSameDT=on
      settings: AttributesFormatString=Criteria=%<Criteria>
  offset1 : Constant  Value=0  OutDataTypeStr=uint16
  offset2 : Constant  Value=0  OutDataTypeStr=uint16
  offset3 : Constant  Value=0  OutDataTypeStr=uint16
  wires:
  Data Type Conversion2/1 -> AEMS_DEM_SETDTR1/4  "uplimit1"
  Data Type Conversion1/1 -> AEMS_DEM_SETDTR1/3  "lowlimit1"
  Data Type Conversion/1 -> AEMS_DEM_SETDTR1/2  "result1"
  DTRId_block1/1 -> AEMS_DEM_SETDTR1/1  "dtrid1"
  upperlimit1/1 -> Limitter3/1
  lowerlimit1/1 -> Limitter2/1
  testresult1/1 -> Limitter1/1
  Sum2/1 -> Data Type Conversion2/1
  Sum1/1 -> Data Type Conversion1/1
  Sum/1 -> Data Type Conversion/1
  Limitter3/1 -> Sum2/2
  offset3/1 -> Sum2/1
  Limitter2/1 -> Sum1/2
  offset2/1 -> Sum1/1
  Limitter1/1 -> Sum/2
  offset1/1 -> Sum/1
  Switch/1 -> AEMS_DEM_SETDTR1/5  "ctrlval1"
  Ctrlval_block1/1 -> Switch/1
  ctrl_flag1/1 -> Switch/2
  Ctrlval_block2/1 -> Switch/3

== system AEMS_Standard_Library/SUB/AEMS_DEM_SET_DTR_8DU/Dem_SetDTR_Call2 ==
  testresult2 : Inport  Interpolate=off
  lowerlimit2 : Inport  Port=2  Interpolate=off
  upperlimit2 : Inport  Port=3  Interpolate=off
  ctrl_flag2 : Inport  Port=4  Interpolate=off
  set_flag2 : EnablePort
      settings: AttributesFormatString=<states=%<StatesWhenEnabling>>
  AEMS_DEM_SETDTR2 : AEMS_Standard_Library/SUB/AEMS_DEM_SETDTR  Tag=[LIB]
      settings: AttributesFormatString=%<MaskType>
  Ctrlval_block1 : Constant  Value=DEM_DTR_CTL_NORMAL  OutDataTypeStr=uint8
  Ctrlval_block2 : Constant  Value=DEM_DTR_CTL_INVISIBLE  OutDataTypeStr=uint8
  DTRId_block2 : Constant  Value=Dem_DtrId2_XXX  OutDataTypeStr=uint16
  Data Type Conversion : DataTypeConversion  OutDataTypeStr=int32  SaturateOnIntegerOverflow=on
  Data Type Conversion1 : DataTypeConversion  OutDataTypeStr=int32  SaturateOnIntegerOverflow=on
  Data Type Conversion2 : DataTypeConversion  OutDataTypeStr=int32  SaturateOnIntegerOverflow=on
  Limitter4 : Saturate  UpperLimit=1  LowerLimit=0
      settings: AttributesFormatString=<limits=%<UpperLimit>/%<LowerLimit>>
  Limitter5 : Saturate  UpperLimit=1  LowerLimit=0
      settings: AttributesFormatString=<limits=%<UpperLimit>/%<LowerLimit>>
  Limitter6 : Saturate  UpperLimit=1  LowerLimit=0
      settings: AttributesFormatString=<limits=%<UpperLimit>/%<LowerLimit>>
  Sum : Sum  OutDataTypeStr=Inherit: Inherit via back propagation  SaturateOnIntegerOverflow=on  InputSameDT=on
  Sum1 : Sum  OutDataTypeStr=Inherit: Inherit via back propagation  SaturateOnIntegerOverflow=on  InputSameDT=on
  Sum2 : Sum  OutDataTypeStr=Inherit: Inherit via back propagation  SaturateOnIntegerOverflow=on  InputSameDT=on
  Switch : Switch  Criteria=u2 ~= 0  ZeroCross=off  InputSameDT=on
      settings: AttributesFormatString=Criteria=%<Criteria>
  offset1 : Constant  Value=0  OutDataTypeStr=uint16
  offset2 : Constant  Value=0  OutDataTypeStr=uint16
  offset3 : Constant  Value=0  OutDataTypeStr=uint16
  wires:
  Data Type Conversion2/1 -> AEMS_DEM_SETDTR2/4  "uplimit2"
  Data Type Conversion1/1 -> AEMS_DEM_SETDTR2/3  "lowlimit2"
  Data Type Conversion/1 -> AEMS_DEM_SETDTR2/2  "result2"
  DTRId_block2/1 -> AEMS_DEM_SETDTR2/1  "dtrid2"
  upperlimit2/1 -> Limitter6/1
  lowerlimit2/1 -> Limitter5/1
  testresult2/1 -> Limitter4/1
  Sum2/1 -> Data Type Conversion2/1
  Sum1/1 -> Data Type Conversion1/1
  Sum/1 -> Data Type Conversion/1
  Limitter6/1 -> Sum2/2
  offset3/1 -> Sum2/1
  Limitter5/1 -> Sum1/2
  offset2/1 -> Sum1/1
  Limitter4/1 -> Sum/2
  offset1/1 -> Sum/1
  Ctrlval_block1/1 -> Switch/1
  ctrl_flag2/1 -> Switch/2
  Ctrlval_block2/1 -> Switch/3
  Switch/1 -> AEMS_DEM_SETDTR2/5  "ctrlval2"

== system AEMS_Standard_Library/SUB/AEMS_DEM_SET_DTR_8DU/Dem_SetDTR_Call3 ==
  testresult3 : Inport  Interpolate=off
  lowerlimit3 : Inport  Port=2  Interpolate=off
  upperlimit3 : Inport  Port=3  Interpolate=off
  ctrl_flag3 : Inport  Port=4  Interpolate=off
  set_flag3 : EnablePort
      settings: AttributesFormatString=<states=%<StatesWhenEnabling>>
  AEMS_DEM_SETDTR3 : AEMS_Standard_Library/SUB/AEMS_DEM_SETDTR  Tag=[LIB]
      settings: AttributesFormatString=%<MaskType>
  Ctrlval_block1 : Constant  Value=DEM_DTR_CTL_NORMAL  OutDataTypeStr=uint8
  Ctrlval_block2 : Constant  Value=DEM_DTR_CTL_INVISIBLE  OutDataTypeStr=uint8
  DTRId_block3 : Constant  Value=Dem_DtrId3_XXX  OutDataTypeStr=uint16
  Data Type Conversion : DataTypeConversion  OutDataTypeStr=int32  SaturateOnIntegerOverflow=on
  Data Type Conversion1 : DataTypeConversion  OutDataTypeStr=int32  SaturateOnIntegerOverflow=on
  Data Type Conversion2 : DataTypeConversion  OutDataTypeStr=int32  SaturateOnIntegerOverflow=on
  Limitter7 : Saturate  UpperLimit=1  LowerLimit=0
      settings: AttributesFormatString=<limits=%<UpperLimit>/%<LowerLimit>>
  Limitter8 : Saturate  UpperLimit=1  LowerLimit=0
      settings: AttributesFormatString=<limits=%<UpperLimit>/%<LowerLimit>>
  Limitter9 : Saturate  UpperLimit=1  LowerLimit=0
      settings: AttributesFormatString=<limits=%<UpperLimit>/%<LowerLimit>>
  Sum : Sum  OutDataTypeStr=Inherit: Inherit via back propagation  SaturateOnIntegerOverflow=on  InputSameDT=on
  Sum1 : Sum  OutDataTypeStr=Inherit: Inherit via back propagation  SaturateOnIntegerOverflow=on  InputSameDT=on
  Sum2 : Sum  OutDataTypeStr=Inherit: Inherit via back propagation  SaturateOnIntegerOverflow=on  InputSameDT=on
  Switch : Switch  Criteria=u2 ~= 0  ZeroCross=off  InputSameDT=on
      settings: AttributesFormatString=Criteria=%<Criteria>
  offset1 : Constant  Value=0  OutDataTypeStr=uint16
  offset2 : Constant  Value=0  OutDataTypeStr=uint16
  offset3 : Constant  Value=0  OutDataTypeStr=uint16
  wires:
  Data Type Conversion2/1 -> AEMS_DEM_SETDTR3/4  "uplimit3"
  Data Type Conversion1/1 -> AEMS_DEM_SETDTR3/3  "lowlimit3"
  Data Type Conversion/1 -> AEMS_DEM_SETDTR3/2  "result3"
  DTRId_block3/1 -> AEMS_DEM_SETDTR3/1  "dtrid3"
  upperlimit3/1 -> Limitter9/1
  lowerlimit3/1 -> Limitter8/1
  testresult3/1 -> Limitter7/1
  Sum2/1 -> Data Type Conversion2/1
  Sum1/1 -> Data Type Conversion1/1
  Sum/1 -> Data Type Conversion/1
  Limitter9/1 -> Sum2/2
  offset3/1 -> Sum2/1
  Limitter8/1 -> Sum1/2
  offset2/1 -> Sum1/1
  Limitter7/1 -> Sum/2
  offset1/1 -> Sum/1
  Ctrlval_block1/1 -> Switch/1
  ctrl_flag3/1 -> Switch/2
  Ctrlval_block2/1 -> Switch/3
  Switch/1 -> AEMS_DEM_SETDTR3/5  "ctrlval3"

== system AEMS_Standard_Library/SUB/AEMS_DEM_SET_DTR_8DU/Dem_SetDTR_Call4 ==
  testresult4 : Inport  Interpolate=off
  lowerlimit4 : Inport  Port=2  Interpolate=off
  upperlimit4 : Inport  Port=3  Interpolate=off
  ctrl_flag4 : Inport  Port=4  Interpolate=off
  set_flag4 : EnablePort
      settings: AttributesFormatString=<states=%<StatesWhenEnabling>>
  AEMS_DEM_SETDTR4 : AEMS_Standard_Library/SUB/AEMS_DEM_SETDTR  Tag=[LIB]
      settings: AttributesFormatString=%<MaskType>
  Ctrlval_block1 : Constant  Value=DEM_DTR_CTL_NORMAL  OutDataTypeStr=uint8
  Ctrlval_block2 : Constant  Value=DEM_DTR_CTL_INVISIBLE  OutDataTypeStr=uint8
  DTRId_block4 : Constant  Value=Dem_DtrId4_XXX  OutDataTypeStr=uint16
  Data Type Conversion : DataTypeConversion  OutDataTypeStr=int32  SaturateOnIntegerOverflow=on
  Data Type Conversion1 : DataTypeConversion  OutDataTypeStr=int32  SaturateOnIntegerOverflow=on
  Data Type Conversion2 : DataTypeConversion  OutDataTypeStr=int32  SaturateOnIntegerOverflow=on
  Limitter10 : Saturate  UpperLimit=1  LowerLimit=0
      settings: AttributesFormatString=<limits=%<UpperLimit>/%<LowerLimit>>
  Limitter11 : Saturate  UpperLimit=1  LowerLimit=0
      settings: AttributesFormatString=<limits=%<UpperLimit>/%<LowerLimit>>
  Limitter12 : Saturate  UpperLimit=1  LowerLimit=0
      settings: AttributesFormatString=<limits=%<UpperLimit>/%<LowerLimit>>
  Sum : Sum  OutDataTypeStr=Inherit: Inherit via back propagation  SaturateOnIntegerOverflow=on  InputSameDT=on
  Sum1 : Sum  OutDataTypeStr=Inherit: Inherit via back propagation  SaturateOnIntegerOverflow=on  InputSameDT=on
  Sum2 : Sum  OutDataTypeStr=Inherit: Inherit via back propagation  SaturateOnIntegerOverflow=on  InputSameDT=on
  Switch : Switch  Criteria=u2 ~= 0  ZeroCross=off  InputSameDT=on
      settings: AttributesFormatString=Criteria=%<Criteria>
  offset1 : Constant  Value=0  OutDataTypeStr=uint16
  offset2 : Constant  Value=0  OutDataTypeStr=uint16
  offset3 : Constant  Value=0  OutDataTypeStr=uint16
  wires:
  Data Type Conversion2/1 -> AEMS_DEM_SETDTR4/4  "uplimit4"
  Data Type Conversion1/1 -> AEMS_DEM_SETDTR4/3  "lowlimit4"
  Data Type Conversion/1 -> AEMS_DEM_SETDTR4/2  "result4"
  DTRId_block4/1 -> AEMS_DEM_SETDTR4/1  "dtrid4"
  upperlimit4/1 -> Limitter12/1
  lowerlimit4/1 -> Limitter11/1
  testresult4/1 -> Limitter10/1
  Sum2/1 -> Data Type Conversion2/1
  Sum1/1 -> Data Type Conversion1/1
  Sum/1 -> Data Type Conversion/1
  Limitter12/1 -> Sum2/2
  offset3/1 -> Sum2/1
  Limitter11/1 -> Sum1/2
  offset2/1 -> Sum1/1
  Limitter10/1 -> Sum/2
  offset1/1 -> Sum/1
  Ctrlval_block1/1 -> Switch/1
  ctrl_flag4/1 -> Switch/2
  Ctrlval_block2/1 -> Switch/3
  Switch/1 -> AEMS_DEM_SETDTR4/5  "ctrlval4"

== system AEMS_Standard_Library/SUB/AEMS_DEM_SET_DTR_8DU/Dem_SetDTR_Call5 ==
  testresult5 : Inport  Interpolate=off
  lowerlimit5 : Inport  Port=2  Interpolate=off
  upperlimit5 : Inport  Port=3  Interpolate=off
  ctrl_flag5 : Inport  Port=4  Interpolate=off
  set_flag5 : EnablePort
      settings: AttributesFormatString=<states=%<StatesWhenEnabling>>
  AEMS_DEM_SETDTR5 : AEMS_Standard_Library/SUB/AEMS_DEM_SETDTR  Tag=[LIB]
      settings: AttributesFormatString=%<MaskType>
  Ctrlval_block1 : Constant  Value=DEM_DTR_CTL_NORMAL  OutDataTypeStr=uint8
  Ctrlval_block2 : Constant  Value=DEM_DTR_CTL_INVISIBLE  OutDataTypeStr=uint8
  DTRId_block5 : Constant  Value=Dem_DtrId5_XXX  OutDataTypeStr=uint16
  Data Type Conversion : DataTypeConversion  OutDataTypeStr=int32  SaturateOnIntegerOverflow=on
  Data Type Conversion1 : DataTypeConversion  OutDataTypeStr=int32  SaturateOnIntegerOverflow=on
  Data Type Conversion2 : DataTypeConversion  OutDataTypeStr=int32  SaturateOnIntegerOverflow=on
  Limitter13 : Saturate  UpperLimit=1  LowerLimit=0
      settings: AttributesFormatString=<limits=%<UpperLimit>/%<LowerLimit>>
  Limitter14 : Saturate  UpperLimit=1  LowerLimit=0
      settings: AttributesFormatString=<limits=%<UpperLimit>/%<LowerLimit>>
  Limitter15 : Saturate  UpperLimit=1  LowerLimit=0
      settings: AttributesFormatString=<limits=%<UpperLimit>/%<LowerLimit>>
  Sum : Sum  OutDataTypeStr=Inherit: Inherit via back propagation  SaturateOnIntegerOverflow=on  InputSameDT=on
  Sum1 : Sum  OutDataTypeStr=Inherit: Inherit via back propagation  SaturateOnIntegerOverflow=on  InputSameDT=on
  Sum2 : Sum  OutDataTypeStr=Inherit: Inherit via back propagation  SaturateOnIntegerOverflow=on  InputSameDT=on
  Switch : Switch  Criteria=u2 ~= 0  ZeroCross=off  InputSameDT=on
      settings: AttributesFormatString=Criteria=%<Criteria>
  offset1 : Constant  Value=0  OutDataTypeStr=uint16
  offset2 : Constant  Value=0  OutDataTypeStr=uint16
  offset3 : Constant  Value=0  OutDataTypeStr=uint16
  wires:
  Data Type Conversion2/1 -> AEMS_DEM_SETDTR5/4  "uplimit5"
  Data Type Conversion1/1 -> AEMS_DEM_SETDTR5/3  "lowlimit5"
  Data Type Conversion/1 -> AEMS_DEM_SETDTR5/2  "result5"
  DTRId_block5/1 -> AEMS_DEM_SETDTR5/1  "dtrid5"
  upperlimit5/1 -> Limitter15/1
  lowerlimit5/1 -> Limitter14/1
  testresult5/1 -> Limitter13/1
  Sum2/1 -> Data Type Conversion2/1
  Sum1/1 -> Data Type Conversion1/1
  Sum/1 -> Data Type Conversion/1
  Limitter15/1 -> Sum2/2
  offset3/1 -> Sum2/1
  Limitter14/1 -> Sum1/2
  offset2/1 -> Sum1/1
  Limitter13/1 -> Sum/2
  offset1/1 -> Sum/1
  Ctrlval_block1/1 -> Switch/1
  ctrl_flag5/1 -> Switch/2
  Ctrlval_block2/1 -> Switch/3
  Switch/1 -> AEMS_DEM_SETDTR5/5  "ctrlval5"

== system AEMS_Standard_Library/SUB/AEMS_DEM_SET_DTR_8DU/Dem_SetDTR_Call6 ==
  testresult6 : Inport  Interpolate=off
  lowerlimit6 : Inport  Port=2  Interpolate=off
  upperlimit6 : Inport  Port=3  Interpolate=off
  ctrl_flag6 : Inport  Port=4  Interpolate=off
  set_flag6 : EnablePort
      settings: AttributesFormatString=<states=%<StatesWhenEnabling>>
  AEMS_DEM_SETDTR6 : AEMS_Standard_Library/SUB/AEMS_DEM_SETDTR  Tag=[LIB]
      settings: AttributesFormatString=%<MaskType>
  Ctrlval_block1 : Constant  Value=DEM_DTR_CTL_NORMAL  OutDataTypeStr=uint8
  Ctrlval_block2 : Constant  Value=DEM_DTR_CTL_INVISIBLE  OutDataTypeStr=uint8
  DTRId_block6 : Constant  Value=Dem_DtrId6_XXX  OutDataTypeStr=uint16
  Data Type Conversion : DataTypeConversion  OutDataTypeStr=int32  SaturateOnIntegerOverflow=on
  Data Type Conversion1 : DataTypeConversion  OutDataTypeStr=int32  SaturateOnIntegerOverflow=on
  Data Type Conversion2 : DataTypeConversion  OutDataTypeStr=int32  SaturateOnIntegerOverflow=on
  Limitter16 : Saturate  UpperLimit=1  LowerLimit=0
      settings: AttributesFormatString=<limits=%<UpperLimit>/%<LowerLimit>>
  Limitter17 : Saturate  UpperLimit=1  LowerLimit=0
      settings: AttributesFormatString=<limits=%<UpperLimit>/%<LowerLimit>>
  Limitter18 : Saturate  UpperLimit=1  LowerLimit=0
      settings: AttributesFormatString=<limits=%<UpperLimit>/%<LowerLimit>>
  Sum : Sum  OutDataTypeStr=Inherit: Inherit via back propagation  SaturateOnIntegerOverflow=on  InputSameDT=on
  Sum1 : Sum  OutDataTypeStr=Inherit: Inherit via back propagation  SaturateOnIntegerOverflow=on  InputSameDT=on
  Sum2 : Sum  OutDataTypeStr=Inherit: Inherit via back propagation  SaturateOnIntegerOverflow=on  InputSameDT=on
  Switch : Switch  Criteria=u2 ~= 0  ZeroCross=off  InputSameDT=on
      settings: AttributesFormatString=Criteria=%<Criteria>
  offset1 : Constant  Value=0  OutDataTypeStr=uint16
  offset2 : Constant  Value=0  OutDataTypeStr=uint16
  offset3 : Constant  Value=0  OutDataTypeStr=uint16
  wires:
  Data Type Conversion2/1 -> AEMS_DEM_SETDTR6/4  "uplimit6"
  Data Type Conversion1/1 -> AEMS_DEM_SETDTR6/3  "lowlimit6"
  Data Type Conversion/1 -> AEMS_DEM_SETDTR6/2  "result6"
  DTRId_block6/1 -> AEMS_DEM_SETDTR6/1  "dtrid6"
  upperlimit6/1 -> Limitter18/1
  lowerlimit6/1 -> Limitter17/1
  testresult6/1 -> Limitter16/1
  Sum2/1 -> Data Type Conversion2/1
  Sum1/1 -> Data Type Conversion1/1
  Sum/1 -> Data Type Conversion/1
  Limitter18/1 -> Sum2/2
  offset3/1 -> Sum2/1
  Limitter17/1 -> Sum1/2
  offset2/1 -> Sum1/1
  Limitter16/1 -> Sum/2
  offset1/1 -> Sum/1
  Ctrlval_block1/1 -> Switch/1
  ctrl_flag6/1 -> Switch/2
  Ctrlval_block2/1 -> Switch/3
  Switch/1 -> AEMS_DEM_SETDTR6/5  "ctrlval6"

== system AEMS_Standard_Library/SUB/AEMS_DEM_SET_DTR_8DU/Dem_SetDTR_Call7 ==
  testresult7 : Inport  Interpolate=off
  lowerlimit7 : Inport  Port=2  Interpolate=off
  upperlimit7 : Inport  Port=3  Interpolate=off
  ctrl_flag7 : Inport  Port=4  Interpolate=off
  set_flag7 : EnablePort
      settings: AttributesFormatString=<states=%<StatesWhenEnabling>>
  AEMS_DEM_SETDTR7 : AEMS_Standard_Library/SUB/AEMS_DEM_SETDTR  Tag=[LIB]
      settings: AttributesFormatString=%<MaskType>
  Ctrlval_block1 : Constant  Value=DEM_DTR_CTL_NORMAL  OutDataTypeStr=uint8
  Ctrlval_block2 : Constant  Value=DEM_DTR_CTL_INVISIBLE  OutDataTypeStr=uint8
  DTRId_block7 : Constant  Value=Dem_DtrId7_XXX  OutDataTypeStr=uint16
  Data Type Conversion : DataTypeConversion  OutDataTypeStr=int32  SaturateOnIntegerOverflow=on
  Data Type Conversion1 : DataTypeConversion  OutDataTypeStr=int32  SaturateOnIntegerOverflow=on
  Data Type Conversion2 : DataTypeConversion  OutDataTypeStr=int32  SaturateOnIntegerOverflow=on
  Limitter19 : Saturate  UpperLimit=1  LowerLimit=0
      settings: AttributesFormatString=<limits=%<UpperLimit>/%<LowerLimit>>
  Limitter20 : Saturate  UpperLimit=1  LowerLimit=0
      settings: AttributesFormatString=<limits=%<UpperLimit>/%<LowerLimit>>
  Limitter21 : Saturate  UpperLimit=1  LowerLimit=0
      settings: AttributesFormatString=<limits=%<UpperLimit>/%<LowerLimit>>
  Sum : Sum  OutDataTypeStr=Inherit: Inherit via back propagation  SaturateOnIntegerOverflow=on  InputSameDT=on
  Sum1 : Sum  OutDataTypeStr=Inherit: Inherit via back propagation  SaturateOnIntegerOverflow=on  InputSameDT=on
  Sum2 : Sum  OutDataTypeStr=Inherit: Inherit via back propagation  SaturateOnIntegerOverflow=on  InputSameDT=on
  Switch : Switch  Criteria=u2 ~= 0  ZeroCross=off  InputSameDT=on
      settings: AttributesFormatString=Criteria=%<Criteria>
  offset1 : Constant  Value=0  OutDataTypeStr=uint16
  offset2 : Constant  Value=0  OutDataTypeStr=uint16
  offset3 : Constant  Value=0  OutDataTypeStr=uint16
  wires:
  Data Type Conversion2/1 -> AEMS_DEM_SETDTR7/4  "uplimit7"
  Data Type Conversion1/1 -> AEMS_DEM_SETDTR7/3  "lowlimit7"
  Data Type Conversion/1 -> AEMS_DEM_SETDTR7/2  "result7"
  DTRId_block7/1 -> AEMS_DEM_SETDTR7/1  "dtrid7"
  upperlimit7/1 -> Limitter21/1
  lowerlimit7/1 -> Limitter20/1
  testresult7/1 -> Limitter19/1
  Sum2/1 -> Data Type Conversion2/1
  Sum1/1 -> Data Type Conversion1/1
  Sum/1 -> Data Type Conversion/1
  Limitter21/1 -> Sum2/2
  offset3/1 -> Sum2/1
  Limitter20/1 -> Sum1/2
  offset2/1 -> Sum1/1
  Limitter19/1 -> Sum/2
  offset1/1 -> Sum/1
  Ctrlval_block1/1 -> Switch/1
  ctrl_flag7/1 -> Switch/2
  Ctrlval_block2/1 -> Switch/3
  Switch/1 -> AEMS_DEM_SETDTR7/5  "ctrlval7"
